simulink library "dhaouadi2013_lib"  (R2025a)
settings: Solver=VariableStepAuto  StartTime=0.0  StopTime=10.0  RelTol=1e-3
settings Model: Creator=nicolls  LastModifiedBy=nicolls

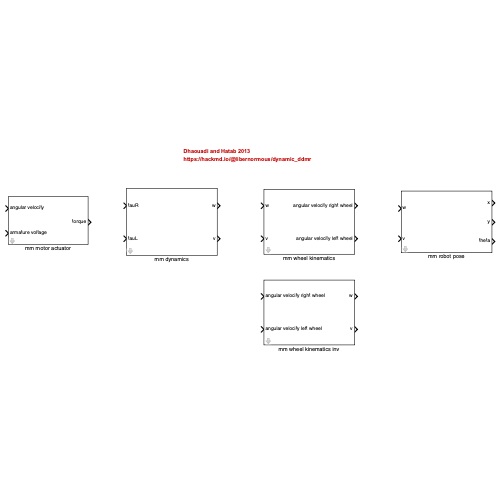
[thumbnail: Simulink's stored preview of the top-level diagram]
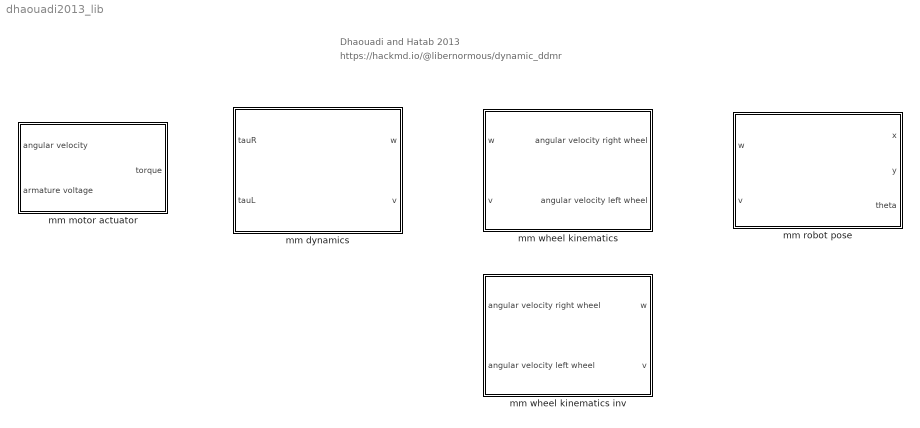
== system dhaouadi2013_lib ==
  note: https://hackmd.io/@libernormous/dynamic_ddmr
  note: Dhaouadi and Hatab 2013
  mm dynamics : Subsystem  mask{m=5, I=2, L=0.05, d=0.02, R=0.025, m_c=5, I_w=0}
      mask prompts: m "m = total robot mass (kg)"; I "I = robot total equivalent inertia (kg.m^2)"; L "L = axle half-length (m)"; d "d = CoM offset from robot center (m)"; R "R = wheel radius (m)"; m_c "m_c = chassis mass without wheels (kg)"; I_w "I_w = wheel intertia (kg.m^2)"
      mask DialogControl Control2 Prompt: See Dhaouadi and Hatab for explanation of parameters.  This block implements their Equation 47.
  mm motor actuator : Subsystem  mask{La=3, Ra=6, Kb=3, N=2, Kt=2}
      mask prompts: La "La = armature winding inductance (H)"; Ra "Ra = armature winding resistance (Ohm)"; Kb "Kb = back emf constant (V/rad/s)"; N "N = gear ratio"; Kt "Kt = torque constant (Nm/A)"
  mm robot pose : Subsystem  mask{x0=0, y0=0, theta0=0}
      mask prompts: x0 "x0 (meters)"; y0 "y0 (meters)"; theta0 "theta0 (rad)"
  mm wheel kinematics : Subsystem  mask{L=0.05, R=0.025}
      mask prompts: L "L = axle half-length (m)"; R "R = wheel radius (m)"
  mm wheel kinematics inv : Subsystem  mask{L=0.05, R=0.025}
      mask prompts: L "L = axle half-length (m)"; R "R = wheel radius (m)"

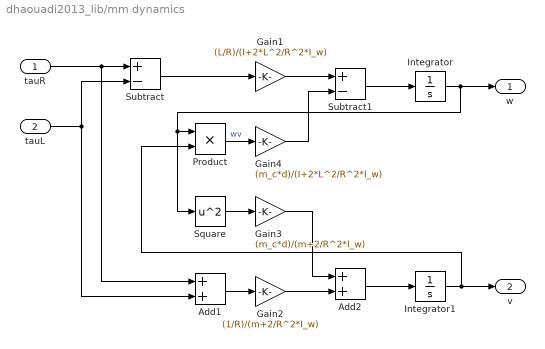
== system dhaouadi2013_lib/mm dynamics ==
  tauR : Inport
  tauL : Inport  Port=2
  Add1 : Sum
  Add2 : Sum
  Gain1 : Gain  Gain=(L/R)/(I+2*L^2/R^2*I_w)
  Gain2 : Gain  Gain=(1/R)/(m+2/R^2*I_w)
  Gain3 : Gain  Gain=(m_c*d)/(m+2/R^2*I_w)
  Gain4 : Gain  Gain=(m_c*d)/(I+2*L^2/R^2*I_w)
  Integrator : Integrator
  Integrator1 : Integrator
  Product : Product
  Square : Math  Operator=square
  Subtract : Sum  Inputs=+-
  Subtract1 : Sum  Inputs=+-
  w : Outport
  v : Outport  Port=2
  wires:
  tauR/1 -> Add1/1, Subtract/1
  tauL/1 -> Add1/2, Subtract/2
  Subtract/1 -> Gain1/1
  Gain1/1 -> Subtract1/1
  Subtract1/1 -> Integrator/1
  Integrator/1 -> w/1, Square/1, Product/1
  Add1/1 -> Gain2/1
  Square/1 -> Gain3/1
  Gain2/1 -> Add2/2
  Gain3/1 -> Add2/1
  Add2/1 -> Integrator1/1
  Integrator1/1 -> v/1, Product/2
  Product/1 -> Gain4/1  "wv"
  Gain4/1 -> Subtract1/2

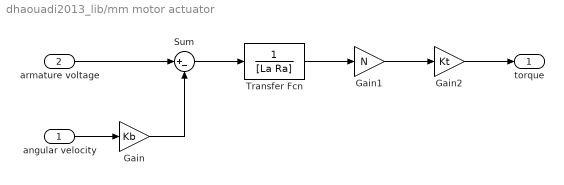
== system dhaouadi2013_lib/mm motor actuator ==
  angular velocity : Inport
  armature voltage : Inport  Port=2
  Gain : Gain  Gain=Kb
  Gain1 : Gain  Gain=N
  Gain2 : Gain  Gain=Kt
  Sum : Sum  Inputs=|+-
  Transfer Fcn : TransferFcn  Denominator=[La Ra]
  torque : Outport
  wires:
  angular velocity/1 -> Gain/1
  Gain/1 -> Sum/2
  armature voltage/1 -> Sum/1
  Sum/1 -> Transfer Fcn/1
  Transfer Fcn/1 -> Gain1/1
  Gain1/1 -> Gain2/1
  Gain2/1 -> torque/1

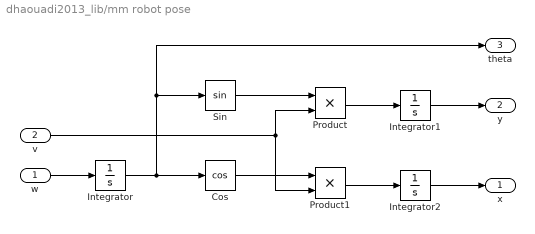
== system dhaouadi2013_lib/mm robot pose ==
  w : Inport
  v : Inport  Port=2
  Cos : Trigonometry  Operator=cos
  Integrator : Integrator  InitialCondition=theta0
  Integrator1 : Integrator  InitialCondition=y0
  Integrator2 : Integrator  InitialCondition=x0
  Product : Product
  Product1 : Product
  Sin : Trigonometry
  x : Outport
  y : Outport  Port=2
  theta : Outport  Port=3
  wires:
  Integrator2/1 -> x/1
  Integrator1/1 -> y/1
  Product1/1 -> Integrator2/1
  Product/1 -> Integrator1/1
  Sin/1 -> Product/1
  Cos/1 -> Product1/1
  v/1 -> Product/2, Product1/2
  Integrator/1 -> theta/1, Sin/1, Cos/1
  w/1 -> Integrator/1

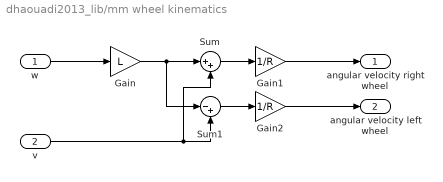
== system dhaouadi2013_lib/mm wheel kinematics ==
  w : Inport
  v : Inport  Port=2
  Gain : Gain  Gain=L
  Gain1 : Gain  Gain=1/R
  Gain2 : Gain  Gain=1/R
  Sum : Sum  Inputs=|++
  Sum1 : Sum  Inputs=|-+
  angular velocity right wheel : Outport
  angular velocity left wheel : Outport  Port=2
  wires:
  w/1 -> Gain/1
  Gain/1 -> Sum1/1, Sum/1
  v/1 -> Sum/2, Sum1/2
  Sum/1 -> Gain1/1
  Sum1/1 -> Gain2/1
  Gain1/1 -> angular velocity right wheel/1
  Gain2/1 -> angular velocity left wheel/1

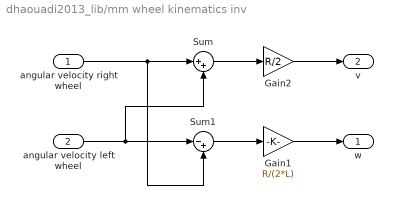
== system dhaouadi2013_lib/mm wheel kinematics inv ==
  angular velocity right wheel : Inport
  angular velocity left wheel : Inport  Port=2
  Gain1 : Gain  Gain=R/(2*L)
  Gain2 : Gain  Gain=R/2
  Sum : Sum  Inputs=|++
  Sum1 : Sum  Inputs=|-+
  w : Outport
  v : Outport  Port=2
  wires:
  Gain1/1 -> w/1
  Gain2/1 -> v/1
  angular velocity right wheel/1 -> Sum/1, Sum1/2
  angular velocity left wheel/1 -> Sum/2, Sum1/1
  Sum1/1 -> Gain1/1
  Sum/1 -> Gain2/1
